simulink model "RespostaDegrau"  (R2020b)
settings: Solver=VariableStepAuto  StartTime=0.0  StopTime=250000  MaxStep=1  RelTol=1e-3
settings Model: Creator=Thiago Saber  LastModifiedBy=Thiago Saber

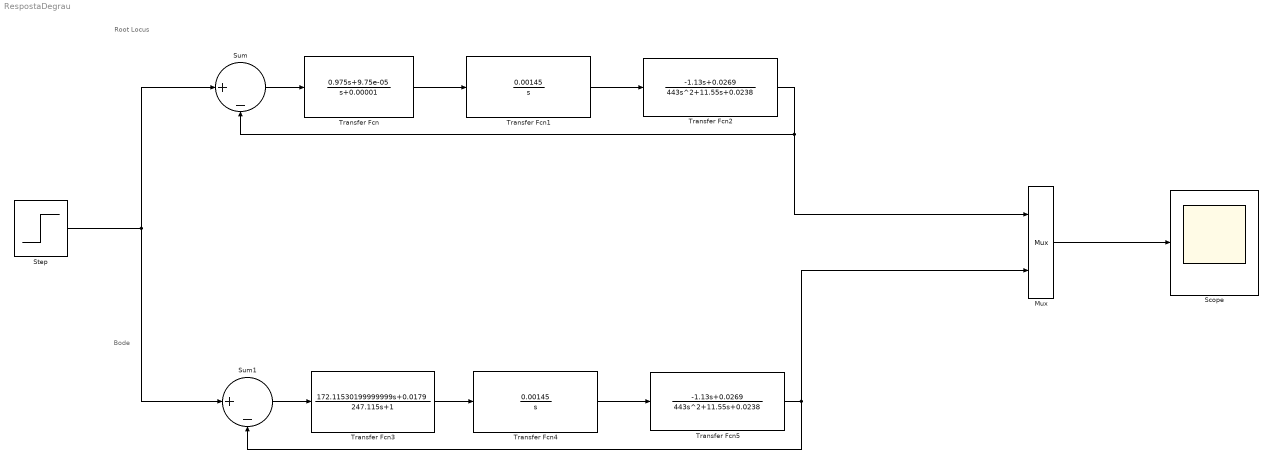
== system RespostaDegrau ==
  note: Bode
  note: Root Locus
  Mux : Mux  Inputs=2
  Scope : Scope
  Step : Step  SampleTime=0
  Sum : Sum  Inputs=|+-
  Sum1 : Sum  Inputs=|+-
  Transfer Fcn : TransferFcn  Numerator=[0.975 9.75e-05]  Denominator=[1 0.00001]
  Transfer Fcn1 : TransferFcn  Numerator=[0.00145]  Denominator=[1 0]
  Transfer Fcn2 : TransferFcn  Numerator=[-1.13 0.0269]  Denominator=[443 11.55 0.0238]
  Transfer Fcn3 : TransferFcn  Numerator=[172.11530199999999 0.0179]  Denominator=[247.115 1]
  Transfer Fcn4 : TransferFcn  Numerator=[0.00145]  Denominator=[1 0]
  Transfer Fcn5 : TransferFcn  Numerator=[-1.13 0.0269]  Denominator=[443 11.55 0.0238]
  wires:
  Sum/1 -> Transfer Fcn/1
  Sum1/1 -> Transfer Fcn3/1
  Transfer Fcn/1 -> Transfer Fcn1/1
  Transfer Fcn1/1 -> Transfer Fcn2/1
  Transfer Fcn2/1 -> Mux/1, Sum/2
  Step/1 -> Sum1/1, Sum/1
  Transfer Fcn3/1 -> Transfer Fcn4/1
  Transfer Fcn4/1 -> Transfer Fcn5/1
  Transfer Fcn5/1 -> Mux/2, Sum1/2
  Mux/1 -> Scope/1
